simulink model "magnetometer"  (R2018b)
settings: Solver=VariableStepAuto  StartTime=0.0  StopTime=10.0  RelTol=1e-3
undefined symbols (not defined in the file or in its folder): magnitude
libraries: simulink x1, vrlib x1, aerolibutil x1
settings Model: Creator=lauren  LastModifiedBy=lauren

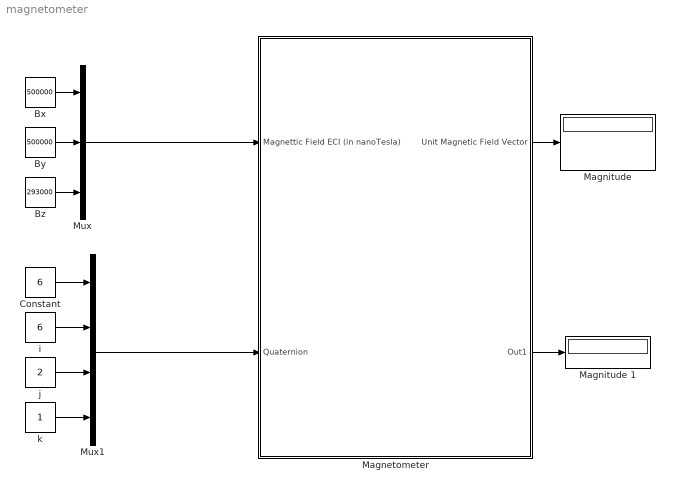
== system magnetometer ==
  " Magnetometer" : Subsystem
  Bx : Constant  Value=500000
  By : Constant  Value=500000
  Bz : Constant  Value=293000
  "Constant " : Constant  Value=6
  "Magnitude " : Display
  Magnitude 1 : Display
  Mux : Mux  Inputs=3
  Mux1 : Mux
  i : Constant  Value=6
  j : Constant  Value=2
  "k " : Constant
  wires:
  Mux/1 -> " Magnetometer"/1(Magnettic Field ECI (in nanoTesla))
  Mux1/1 -> " Magnetometer"/2("Quaternion ")
  " Magnetometer"/1(Unit Magnetic Field Vector) -> "Magnitude "/1
  By/1 -> Mux/2
  Bx/1 -> Mux/1
  Bz/1 -> Mux/3
  i/1 -> Mux1/2
  "Constant "/1 -> Mux1/1
  j/1 -> Mux1/3
  "k "/1 -> Mux1/4
  " Magnetometer"/2(Out1) -> Magnitude 1/1

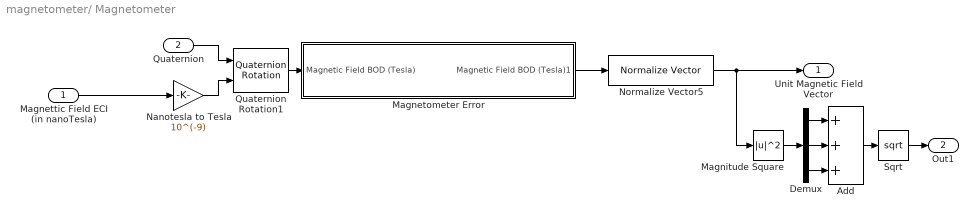
== system magnetometer/ Magnetometer ==
  Magnettic Field ECI (in nanoTesla) : Inport
  "Quaternion " : Inport  Port=2
  Add : Sum  Inputs=3
  Demux : Demux  Outputs=3
  Magnetometer Error : Subsystem
  Magnitude Square : Math  Operator=magnitude^2  RndMeth=Zero  SaturateOnIntegerOverflow=on
  Nanotesla to Tesla : Gain  Gain=10^(-9)
  Normalize Vector5 : vrlib/Utilities/Normalize Vector  maxzero=0
      settings: SourceProductName=Simulink 3D Animation  SourceProductBaseCode=VR
  Quaternion Rotation1 : aerolibutil/Quaternion Rotation
  Sqrt : Sqrt  SaturateOnIntegerOverflow=on
  Unit Magnetic Field Vector : Outport
  Out1 : Outport  Port=2
  wires:
  Magnettic Field ECI (in nanoTesla)/1 -> Nanotesla to Tesla/1
  Magnetometer Error/1("Magnetic Field BOD (Tesla)1 ") -> Normalize Vector5/1
  Normalize Vector5/1 -> Magnitude Square/1, Unit Magnetic Field Vector/1
  "Quaternion "/1 -> Quaternion Rotation1/1
  Nanotesla to Tesla/1 -> Quaternion Rotation1/2
  Quaternion Rotation1/1 -> Magnetometer Error/1(Magnetic Field BOD (Tesla))
  Magnitude Square/1 -> Demux/1
  Demux/1 -> Add/1
  Demux/2 -> Add/2
  Demux/3 -> Add/3
  Add/1 -> Sqrt/1
  Sqrt/1 -> Out1/1

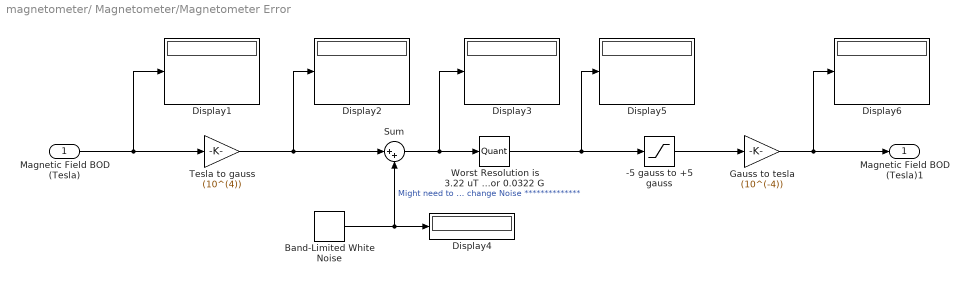
== system magnetometer/ Magnetometer/Magnetometer Error ==
  Magnetic Field BOD (Tesla) : Inport
  -5 gauss to +5 gauss : Saturate  UpperLimit=5  LowerLimit=-5
  Band-Limited White Noise : simulink/Sources/Band-Limited White Noise  Cov=0.1  Ts=0.1  seed=[23341]
  Display{1..6} (6 alike) : Display
  Gauss to tesla : Gain  Gain=(10^(-4))
  Sum : Sum  Inputs=|++
  Tesla to gauss : Gain  Gain=(10^(4))
  Worst Resolution is 3.22 uT or 0.0322 G : Quantizer  QuantizationInterval=0.0322
  "Magnetic Field BOD (Tesla)1 " : Outport
  wires:
  -5 gauss to +5 gauss/1 -> Gauss to tesla/1
  Sum/1 -> Display3/1, Worst Resolution is 3.22 uT or 0.0322 G/1
  Tesla to gauss/1 -> Display2/1, Sum/1
  Band-Limited White Noise/1 -> Display4/1, Sum/2  "Might need to  change Noise **************"
  Worst Resolution is 3.22 uT or 0.0322 G/1 -> Display5/1, -5 gauss to +5 gauss/1
  Magnetic Field BOD (Tesla)/1 -> Display1/1, Tesla to gauss/1
  Gauss to tesla/1 -> Display6/1, "Magnetic Field BOD (Tesla)1 "/1
